simulink model "a622"  (R2019b)
settings: Solver=VariableStepAuto  StartTime=0.0  StopTime=300  RelTol=1e-3
libraries: simulink x1
settings Model: Creator=ovi  LastModifiedBy=ovi

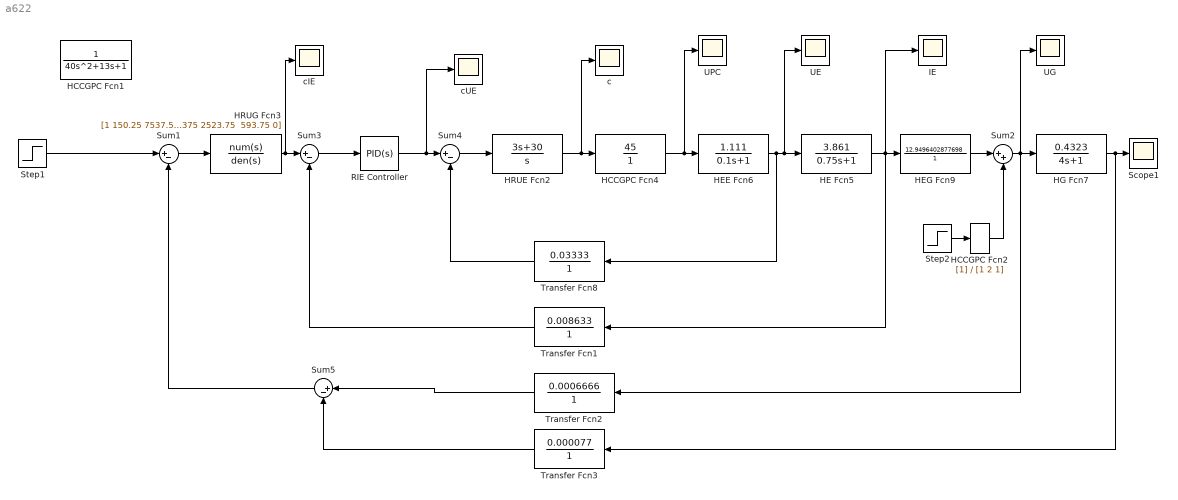
== system a622 ==
  HCCGPC Fcn1 : TransferFcn  Denominator=[40 13 1]
  HCCGPC Fcn2 : TransferFcn
  HCCGPC Fcn4 : TransferFcn  Numerator=[45]  Denominator=[1]
  HE Fcn5 : TransferFcn  Numerator=[3.861]  Denominator=[0.75 1]
  HEE Fcn6 : TransferFcn  Numerator=[1.111]  Denominator=[0.1 1]
  HEG Fcn9 : TransferFcn  Numerator=[12.9496402877698]  Denominator=[1]
  HG Fcn7 : TransferFcn  Numerator=[0.4323]  Denominator=[4 1]
  HRUE Fcn2 : TransferFcn  Numerator=[3 30]  Denominator=[1 0]
  HRUG Fcn3 : TransferFcn  Numerator=[1 150.25 7537.5 126875 31250]  Denominator="[1 100.2375 2523.75  593.75 0]"
  IE : Scope
  RIE Controller : simulink/Continuous/PID Controller  Controller=PID  Form=Parallel  TimeDomain=Continuous-time  SampleTime=-1  IntegratorMethod=Forward Euler  FilterMethod=Forward Euler  ControllerParametersSource=internal  P=38.5  I=50  D=0.75  UseFilter=on  N=2  TunerSelectOption=Transfer Function Based (PID Tuner App)  InitialConditionSource=internal  InitialConditionForIntegrator=0  InitialConditionForFilter=0  DifferentiatorICPrevScaledInput=0  ExternalReset=none  TrackingMode=off  Kt=1  LimitOutput=off  UpperSaturationLimit=inf  LowerSaturationLimit=-inf  LinearizeAsGain=on  AntiWindupMode=none  Kb=1  POutMin=[]  POutMax=[]  IOutMin=[]  IOutMax=[]  DOutMin=[]  DOutMax=[]  NOutMin=[]  NOutMax=[]  SumOutMin=[]  SumOutMax=[]  SaturationOutMin=[]  SaturationOutMax=[]  PParamMin=[]  PParamMax=[]  IParamMin=[]  IParamMax=[]  DParamMin=[]  DParamMax=[]  NParamMin=[]  NParamMax=[]  KbParamMin=[]  KbParamMax=[]  KtParamMin=[]  KtParamMax=[]  KbOutMin=[]  KbOutMax=[]  KtOutMin=[]  KtOutMax=[]  IntegratorOutMin=[]  IntegratorOutMax=[]  FilterOutMin=[]  FilterOutMax=[]  SumI1OutMin=[]  SumI1OutMax=[]  SumI2OutMin=[]  SumI2OutMax=[]  SumI3OutMin=[]  SumI3OutMax=[]  SumI4OutMin=[]  SumI4OutMax=[]  SumDOutMin=[]  SumDOutMax=[]  DifferentiatorOutMin=[]  DifferentiatorOutMax=[]  FilterDiffOutCoefMin=[]  FilterDiffOutCoefMax=[]  ReciprocalOutMin=[]  ReciprocalOutMax=[]  SumDenOutMin=[]  SumDenOutMax=[]  SumNumOutMin=[]  SumNumOutMax=[]  DivideOutMin=[]  DivideOutMax=[]  IntegratorContinuousStateAttributes=''  IntegratorStateMustResolveToSignalObject=off  IntegratorRTWStateStorageClass=Auto  FilterContinuousStateAttributes=''  FilterStateMustResolveToSignalObject=off  FilterRTWStateStorageClass=Auto  ParallelPVariant=InternalParameters  IdealPVariant=Disabled  IVariant=InternalParameters  DVariant=InternalParameters  IntegratorVariant=Continuous  SatVariant=Disabled  AWVariant=Passthrough  PCopyVariant=Disabled  TRVariant=Disabled  FdbkBlocksVariant=Forward  IdealPFdbkVariant=Disabled  SatFdbkVariant=Disabled  DerivativeFilterVariant=ContFilter  NVariant=InternalParameters  NCopyVariant=Disabled  FilterICVariant=InternalICsFilter  IntegratorICVariant=InternalICs  ExternalResetVariant=Disabled  TRSumVariant=Passthrough  SumFdbkVariant=Disabled  SumVariant=Sum_PID
  Scope1 : Scope
  Step1 : Step  After=9.5  SampleTime=0
  Step2 : Step  Time=80  After=-1000  SampleTime=0
  Sum{1,3..5} (4 alike) : Sum  Inputs=|+-
  Sum2 : Sum  Inputs=|++
  Transfer Fcn1 : TransferFcn  Numerator=0.008633  Denominator=1
  Transfer Fcn2 : TransferFcn  Numerator=0.0006666  Denominator=1
  Transfer Fcn3 : TransferFcn  Numerator=0.000077  Denominator=1
  Transfer Fcn8 : TransferFcn  Numerator=[0.03333]  Denominator=1
  UE : Scope
  UG : Scope
  UPC : Scope
  c : Scope
  cIE : Scope
  cUE : Scope
  wires:
  Sum1/1 -> HRUG Fcn3/1
  Sum3/1 -> RIE Controller/1
  HRUG Fcn3/1 -> cIE/1, Sum3/1
  Sum4/1 -> HRUE Fcn2/1
  RIE Controller/1 -> cUE/1, Sum4/1
  HRUE Fcn2/1 -> c/1, HCCGPC Fcn4/1
  HEE Fcn6/1 -> Transfer Fcn8/1, UE/1, HE Fcn5/1
  HCCGPC Fcn4/1 -> UPC/1, HEE Fcn6/1
  Sum2/1 -> UG/1, Transfer Fcn2/1, HG Fcn7/1
  Step2/1 -> HCCGPC Fcn2/1
  HG Fcn7/1 -> Transfer Fcn3/1, Scope1/1
  HEG Fcn9/1 -> Sum2/1
  HE Fcn5/1 -> IE/1, Transfer Fcn1/1, HEG Fcn9/1
  Transfer Fcn8/1 -> Sum4/2
  Transfer Fcn1/1 -> Sum3/2
  Transfer Fcn2/1 -> Sum5/1
  Transfer Fcn3/1 -> Sum5/2
  Sum5/1 -> Sum1/2
  HCCGPC Fcn2/1 -> Sum2/2
  Step1/1 -> Sum1/1
